simulink model "untitled1"  (R2023b)
settings: Solver=FixedStepAuto  StartTime=0.0  StopTime=9  FixedStep=1e-3  RelTol=1e-3
values from neighbouring files (symbols this model uses):
  denc = [0.01 1]    [untitled.m]
  denc1 = [0.01 1]    [untitled.m]
  denx = [0.1 1 ]    [untitled.m]
  deny = [0.75 1 ]    [untitled.m]
  numc = [0.1 1]    [untitled.m]
  numc1 = [0.4 1]    [untitled.m]
  numx = [2]    [untitled.m]
  numy = [3]    [untitled.m]
libraries: simulink x4
settings Model: Creator=paul-andreipintea  LastModifiedBy=paul-andreipintea

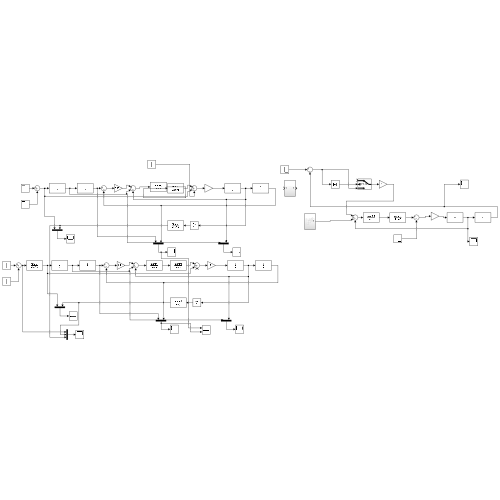
[thumbnail: Simulink's stored preview of the top-level diagram]
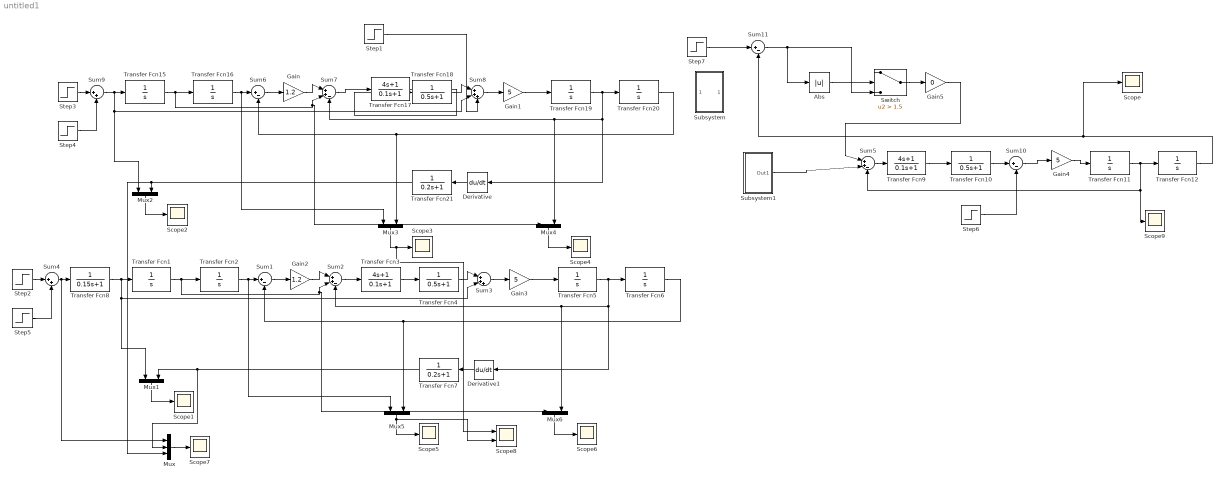
== system untitled1 ==
  Abs : Abs  SaturateOnIntegerOverflow=off
  Derivative : Derivative
  Derivative1 : Derivative
  Gain : Gain  Gain=1.2
  Gain1 : Gain  Gain=5
  Gain2 : Gain  Gain=1.2
  Gain3 : Gain  Gain=5
  Gain4 : Gain  Gain=5
  Gain5 : Gain  Gain=0
  Mux : Mux  Inputs=3
  Mux{1..6} (6 alike) : Mux  Inputs=2
  Scope{,1..7,9} (9 alike) : Scope
  Scope8 : Scope  NumInputPorts=2
  Step1 : Step  Time=7  After=-1  SampleTime=0
  Step2 : Step  Time=4  Before=1  After=0  SampleTime=0
  Step3 : Step  Time=4  Before=1  After=0  SampleTime=0
  Step4 : Step  Time=5  After=-1  SampleTime=0
  Step5 : Step  Time=5  After=-1  SampleTime=0
  Step6 : Step  Time=7  After=-1  SampleTime=0
  Step7 : Step  Time=7  After=-1  SampleTime=0
  Subsystem : Subsystem
  Subsystem1 : Subsystem
  Sum{1,6,10..11} (4 alike) : Sum  Inputs=|+-
  Sum2 : Sum  Inputs=|++-
  Sum3 : Sum  Inputs=|+++
  Sum4 : Sum  Inputs=|++
  Sum5 : Sum  Inputs=|++-
  Sum7 : Sum  Inputs=|++-
  Sum8 : Sum  Inputs=|+++
  Sum9 : Sum  Inputs=|++
  Switch : Switch  Criteria=u2 > Threshold  Threshold=1.5  SaturateOnIntegerOverflow=off  InputSameDT=off
  Transfer Fcn{1..2,5..6,11..12,15..16,19..20} (10 alike) : TransferFcn  Denominator=[1 0]
  Transfer Fcn10 : TransferFcn  Numerator=[ 1]  Denominator=[0.5 1]
  Transfer Fcn17 : TransferFcn  Numerator=[4 1]  Denominator=[0.1 1]
  Transfer Fcn18 : TransferFcn  Numerator=[ 1]  Denominator=[0.5 1]
  Transfer Fcn21 : TransferFcn  Numerator=[ 1]  Denominator=[0.2 1]
  Transfer Fcn3 : TransferFcn  Numerator=[4 1]  Denominator=[0.1 1]
  Transfer Fcn4 : TransferFcn  Numerator=[ 1]  Denominator=[0.5 1]
  Transfer Fcn7 : TransferFcn  Numerator=[ 1]  Denominator=[0.2 1]
  Transfer Fcn8 : TransferFcn  Denominator=[0.15 1]
  Transfer Fcn9 : TransferFcn  Numerator=[4 1]  Denominator=[0.1 1]
  wires:
  Transfer Fcn15/1 -> Mux4/1, Sum7/2, Transfer Fcn16/1
  Transfer Fcn16/1 -> Mux3/1, Sum6/1
  Sum6/1 -> Gain/1
  Gain/1 -> Sum7/1
  Sum7/1 -> Transfer Fcn17/1
  Transfer Fcn17/1 -> Transfer Fcn18/1
  Transfer Fcn18/1 -> Sum8/1
  Sum8/1 -> Gain1/1
  Transfer Fcn19/1 -> Derivative/1, Sum7/3, Mux4/2, Transfer Fcn20/1
  Gain1/1 -> Transfer Fcn19/1
  Transfer Fcn20/1 -> Sum6/2, Mux3/2
  Step3/1 -> Sum9/1
  Step4/1 -> Sum9/2
  Sum9/1 -> Mux2/1, Sum8/2, Transfer Fcn15/1
  Derivative/1 -> Transfer Fcn21/1
  Transfer Fcn21/1 -> Mux/3, Mux2/2
  Mux2/1 -> Scope2/1
  Mux3/1 -> Scope8/1, Scope3/1
  Mux4/1 -> Scope4/1
  Mux6/1 -> Scope6/1
  Mux1/1 -> Scope1/1
  Transfer Fcn7/1 -> Mux/2, Mux1/2
  Derivative1/1 -> Transfer Fcn7/1
  Transfer Fcn8/1 -> Transfer Fcn1/1, Sum3/2, Mux1/1
  Step5/1 -> Sum4/2
  Step2/1 -> Sum4/1
  Transfer Fcn6/1 -> Mux5/2, Sum1/2
  Gain3/1 -> Transfer Fcn5/1
  Transfer Fcn5/1 -> Transfer Fcn6/1, Mux6/2, Sum2/3, Derivative1/1
  Sum3/1 -> Gain3/1
  Transfer Fcn4/1 -> Sum3/1
  Transfer Fcn3/1 -> Transfer Fcn4/1
  Sum2/1 -> Transfer Fcn3/1
  Gain2/1 -> Sum2/1
  Sum1/1 -> Gain2/1
  Transfer Fcn2/1 -> Sum1/1, Mux5/1
  Transfer Fcn1/1 -> Transfer Fcn2/1, Sum2/2, Mux6/1
  Sum4/1 -> Mux/1, Transfer Fcn8/1
  Mux/1 -> Scope7/1
  Mux5/1 -> Scope8/2, Scope5/1
  Step1/1 -> Sum8/3
  Gain4/1 -> Transfer Fcn11/1
  Transfer Fcn11/1 -> Transfer Fcn12/1, Scope9/1, Sum5/3
  Sum10/1 -> Gain4/1
  Transfer Fcn10/1 -> Sum10/1
  Transfer Fcn9/1 -> Transfer Fcn10/1
  Sum5/1 -> Transfer Fcn9/1
  Step6/1 -> Sum10/2
  Subsystem1/1(Out1) -> Sum5/2
  Step7/1 -> Sum11/1
  Abs/1 -> Switch/2
  Sum11/1 -> Switch/3, Abs/1
  Switch/1 -> Gain5/1
  Gain5/1 -> Sum5/1
  Transfer Fcn12/1 -> Scope/1, Sum11/2

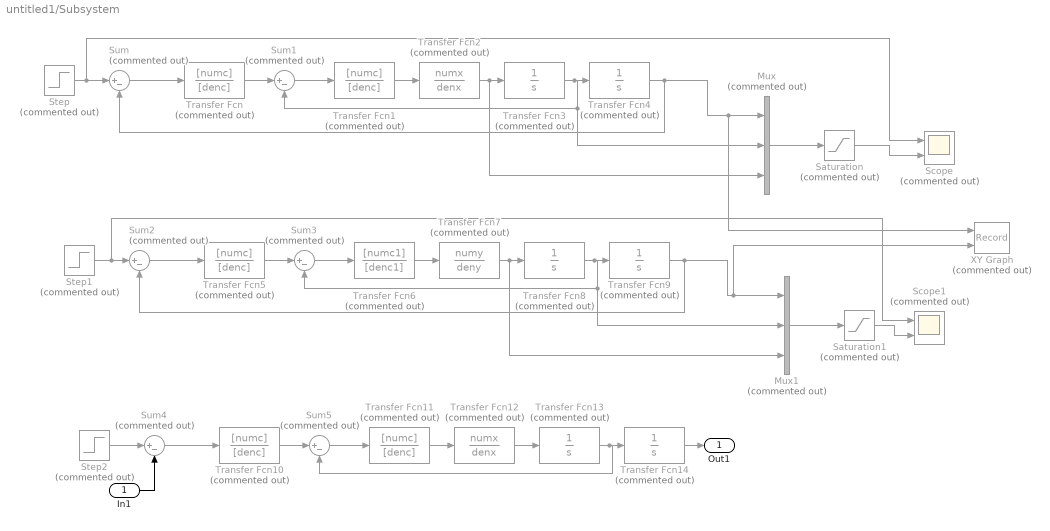
== system untitled1/Subsystem ==
  In1 : Inport
  Mux : Mux  Commented=on  Inputs=3
  Mux1 : Mux  Commented=on  Inputs=3
  Saturation : Saturate  Commented=on  UpperLimit=inf  LowerLimit=-inf
  Saturation1 : Saturate  Commented=on  UpperLimit=inf  LowerLimit=-inf
  Scope : Scope  Commented=on  NumInputPorts=2
  Scope1 : Scope  Commented=on  NumInputPorts=2
  Step : Step  Commented=on  Time=17  Before=40  After=80  SampleTime=0
  Step1 : Step  Commented=on  Before=60  After=60  SampleTime=0
  Step2 : Step  Commented=on  Time=17  Before=40  After=80  SampleTime=0
  Sum{,1..5} (6 alike) : Sum  Commented=on  Inputs=|+-
  Transfer Fcn{,1,5,10..11} (5 alike) : TransferFcn  Commented=on  Numerator=[numc]  Denominator=[denc]
  Transfer Fcn12 : TransferFcn  Commented=on  Numerator=numx  Denominator=denx
  Transfer Fcn{3..4,8..9,13..14} (6 alike) : TransferFcn  Commented=on  Denominator=[1 0]
  Transfer Fcn2 : TransferFcn  Commented=on  Numerator=numx  Denominator=denx
  Transfer Fcn6 : TransferFcn  Commented=on  Numerator=[numc1]  Denominator=[denc1]
  Transfer Fcn7 : TransferFcn  Commented=on  Numerator=numy  Denominator=deny
  XY Graph : Record  Commented=on  FileSettingsInternal="{\"entries\":[{\"content\":{\"excelSettings\":{\"content\":{},\"type\":\"Streamout.ExcelSettings\"}},\"type\":\"Streamout.FileSettingStorage\",\"uuid\":\"\"}],\"packageUris\":[\"http:\\/\\/schema.mathworks.com\\/mf0\\/streamout_blocks\\/R2020a\"],\"version\":\"1.0\"}"  Layout=[1 1]  SignalsInternal="{\"entries\":[{\"content\":{\"signals\":[{\"content\":{\"blockPath\":[],\"dimensions\":[1],\"domain\":\"\",\"lineColor\":\"#a2142f\",\"plots\":[1],\"port\":1,\"sid\":[\"\"],\"signalID\":29,\"signalName\":\"Transfer Fcn4\"},\"type\":\"RecordBlkView.Signal\",\"uuid\":\"\"},{\"content\":{\"blockPath\":[],\"dimensions\":[1],\"domain\":\"\",\"lineColor\":\"#139fff\",\"plots\":[1],\"port\":2,\"sid\":[\"\"],\"signalID\":33,\"signalName\":\"Transfer Fcn9\"},\"type\":\"RecordBlkView.Signal\",\"uuid\":\"\"}]},\"type\":\"RecordBlkView.InputSignals\",\"uuid\":\"\"}],\"packageUris\":[\"http:\\/\\/schema.mathworks.com\\/mf0\\/streamout_blocks\\/R2020a\"],\"version\":\"1.0\"}"  VisualizationBindings="{\"xyplotplugin\":{\"info\":[{\"series\":[{\"bindingParametersList\":[{\"parameter\":\"X-Axis\",\"signalID\":29,\"signalName\":\"Transfer Fcn4\"},{\"parameter\":\"Y-Axis\",\"signalID\":33,\"signalName\":\"Transfer Fcn9\"}],\"seriesID\":43623}],\"subplotID\":1}]}}"  CompatibilityTag=XY
  Out1 : Outport
  wires:
  In1/1 -> Sum4/2
  Transfer Fcn14/1 -> Out1/1
  Step2/1 -> Sum4/1
  Transfer Fcn10/1 -> Sum5/1
  Transfer Fcn5/1 -> Sum3/1
  Transfer Fcn6/1 -> Transfer Fcn7/1
  Transfer Fcn/1 -> Sum1/1
  Sum3/1 -> Transfer Fcn6/1
  Transfer Fcn2/1 -> Mux/3, Transfer Fcn3/1
  Mux1/1 -> Saturation1/1
  Sum2/1 -> Transfer Fcn5/1
  Transfer Fcn4/1 -> Sum/2, XY Graph/1, Mux/1
  Sum5/1 -> Transfer Fcn11/1
  Saturation1/1 -> Scope1/2
  Step/1 -> Scope/1, Sum/1
  Transfer Fcn8/1 -> Mux1/2, Sum3/2, Transfer Fcn9/1
  Transfer Fcn11/1 -> Transfer Fcn12/1
  Transfer Fcn3/1 -> Mux/2, Sum1/2, Transfer Fcn4/1
  Sum4/1 -> Transfer Fcn10/1
  Mux/1 -> Saturation/1
  Transfer Fcn13/1 -> Sum5/2, Transfer Fcn14/1
  Transfer Fcn9/1 -> Sum2/2, XY Graph/2, Mux1/1
  Transfer Fcn12/1 -> Transfer Fcn13/1
  Transfer Fcn7/1 -> Mux1/3, Transfer Fcn8/1
  Step1/1 -> Scope1/1, Sum2/1
  Saturation/1 -> Scope/2
  Transfer Fcn1/1 -> Transfer Fcn2/1
  Sum/1 -> Transfer Fcn/1
  Sum1/1 -> Transfer Fcn1/1

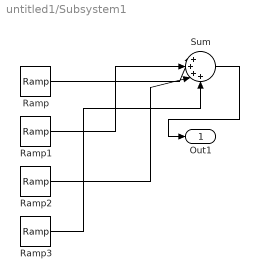
== system untitled1/Subsystem1 ==
  Ramp : simulink/Sources/Ramp  slope=1  start=0  InitialOutput=0
  Ramp1 : simulink/Sources/Ramp  slope=-1  start=4  InitialOutput=0
  Ramp2 : simulink/Sources/Ramp  slope=-1  start=5  InitialOutput=0
  Ramp3 : simulink/Sources/Ramp  slope=1  start=9  InitialOutput=0
  Sum : Sum  Inputs=|++++
  Out1 : Outport
  wires:
  Sum/1 -> Out1/1
  Ramp/1 -> Sum/1
  Ramp1/1 -> Sum/2
  Ramp2/1 -> Sum/3
  Ramp3/1 -> Sum/4
